simulink model "acs323_m5"  (R2025b)
settings: Solver=ode45  StartTime=0.0  StopTime=300  MaxStep=1  RelTol=1e-3  AbsTol=1e-3  EnableMultiTasking=on
libraries: fuzblock x1, simulink_need_slupdate x1
settings Model: ExtModeTrigMode=oneshot  ExtModeArmWhenConnect=off  Creator=uos  LastModifiedBy=willnatsan
settings SolverCC: AutoScaleAbsTol=off  AlgebraicLoopSolver=TrustRegion
settings DataIOCC: SaveFormat=Array  SignalLoggingSaveFormat=ModelDataLogs  SaveOutput=off  SaveTime=off  ReturnWorkspaceOutputs=off  SignalLoggingName=sigsOut
settings OptimizationCC: BooleanDataType=off  ReuseModelBlockBuffer=off
settings DebuggingCC: SaveWithParameterizedLinksMsg=none  UnderspecifiedInitializationDetection=Classic  MergeDetectMultiDrivingBlocksExec=none  SignalResolutionControl=TryResolveAllWithWarning  MultiTaskDSMMsg=warning  MultiTaskCondExecSysMsg=none  UnconnectedInputMsg=warning  UnconnectedOutputMsg=warning  UnconnectedLineMsg=warning  ArithmeticOperatorsInVariantConditions=warning
settings HardwareCC: ProdBitPerPointer=32.0  ProdBitPerSizeT=32.0  ProdBitPerPtrDiffT=32.0  ProdLargestAtomicFloat=None  ProdIntDivRoundTo=Undefined  ProdEndianess=Unspecified  ProdWordSize=32.0  ProdHWDeviceType=32-bit Generic  TargetUnknown=on
settings ModelReferenceCC: EnableRefExpFcnMdlSchedulingChecks=on  PropagateSignalLabelsOutOfModel=off
settings SFSimCC: SimUseLocalCustomCode=off  CustomCodeUndefinedFunction=UseInterfaceOnly
settings RTWCC: RTWUseLocalCustomCode=off  GPUComputeCapability=3.5  DLArmComputeVersion=19.05
settings GRTTargetCC: TargetLangStandard=C89/C90 (ANSI)  CombineOutputUpdateFcns=off  GRTInterface=on
settings ConfigComp: CovMetricSettings=dw  CovSaveCumulativeToWorkspaceVar=on  CovSaveSingleToWorkspaceVar=on  CovExternalEMLEnable=off

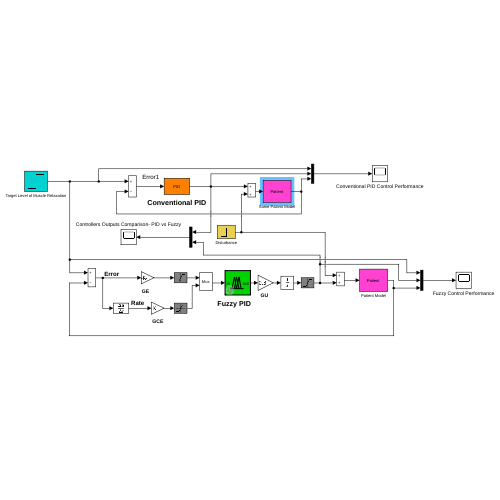
[thumbnail: Simulink's stored preview of the top-level diagram]
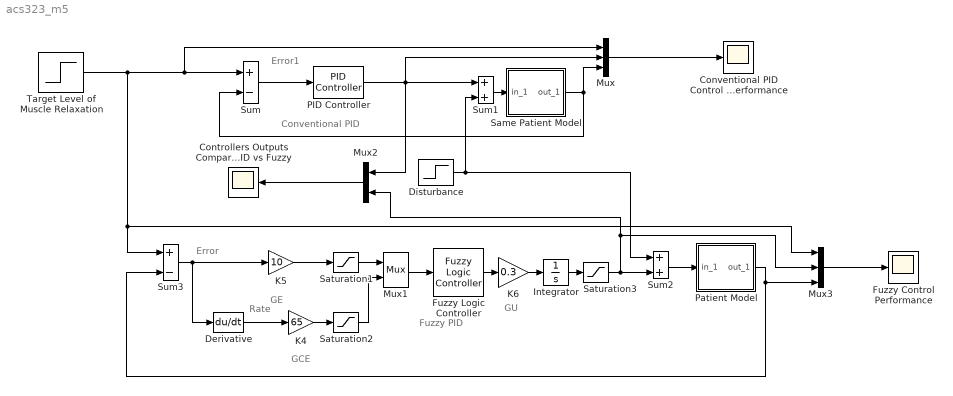
== system acs323_m5 ==
  note: Fuzzy PID
  note: Conventional PID
  note: GE
  note: GCE
  note: GU
  note: Error
  note: Rate
  note: Error1
  Controllers Outputs Comparison- PID vs Fuzzy : Scope
      settings: ActiveDisplayYMinimum=0  ActiveDisplayYMaximum=1.2
  Conventional PID Control Performance : Scope
      settings: ActiveDisplayYMinimum=0.24324  ActiveDisplayYMaximum=0.97781  DataLoggingVariableName=ScopeData2
  Derivative : Derivative
  Disturbance : Step  Time=150  After=0.2  SampleTime=0
  Fuzzy Control Performance : Scope
      settings: ActiveDisplayYMinimum=-0.125  ActiveDisplayYMaximum=1.125
  Fuzzy Logic Controller : fuzblock/Fuzzy Logic  Controller  FIS="\"patient.fis\""  OutputSampleNumber=101  DataType=double  UseLookupTable=off  NumBreakpoints=10  FuzzifiedInputs=off  RuleFiringStrengths=off  RuleOutputs=off  AggregatedOutputs=off  SimulateUsing=Interpreted execution  OutOfRangeInputValueMessage=warning  NoRuleFiredMessage=warning  EmptyOutputFuzzySetMessage=warning
  Integrator : Integrator
  K4 : Gain  Gain=65  SaturateOnIntegerOverflow=on  OutDataTypeStr=Inherit: Same as input  ParamDataTypeStr=Inherit: Same as input
  K5 : Gain  Gain=10  SaturateOnIntegerOverflow=on  OutDataTypeStr=Inherit: Same as input  ParamDataTypeStr=Inherit: Same as input
  K6 : Gain  Gain=0.3  SaturateOnIntegerOverflow=on  OutDataTypeStr=Inherit: Same as input  ParamDataTypeStr=Inherit: Same as input
  Mux : Mux  Inputs=3
  Mux1 : Mux  Inputs=2
  Mux2 : Mux  Inputs=2
  Mux3 : Mux  Inputs=3
  PID Controller : simulink_need_slupdate/PID Controller  P=0.80  I=0.04  D=0
  Patient Model : Subsystem
      mask Display: disp('Patient')
  Same Patient Model : Subsystem
      mask Display: disp('Patient')
  Saturation1 : Saturate  UpperLimit=1  LowerLimit=-1
  Saturation2 : Saturate  UpperLimit=1  LowerLimit=-1
  Saturation3 : Saturate  UpperLimit=1  LowerLimit=0
  Sum : Sum  Inputs=+-  InputSameDT=on  SaturateOnIntegerOverflow=on  OutDataTypeStr=Inherit: Same as first input
  Sum1 : Sum  InputSameDT=on  SaturateOnIntegerOverflow=on  OutDataTypeStr=Inherit: Same as first input
  Sum2 : Sum  InputSameDT=on  SaturateOnIntegerOverflow=on  OutDataTypeStr=Inherit: Same as first input
  Sum3 : Sum  Inputs=+-  InputSameDT=on  SaturateOnIntegerOverflow=on  OutDataTypeStr=Inherit: Same as first input
  Target Level of Muscle Relaxation : Step  Time=0  After=0.8  SampleTime=0
  wires:
  Sum/1 -> PID Controller/1
  Saturation2/1 -> Mux1/2
  Saturation1/1 -> Mux1/1
  Mux1/1 -> Fuzzy Logic Controller/1
  Target Level of Muscle Relaxation/1 -> Sum/1, Mux/1, Mux3/1, Sum3/1
  Sum1/1 -> Same Patient Model/1(in_1)
  Sum2/1 -> Patient Model/1(in_1)
  Saturation3/1 -> Sum2/2, Mux3/2, Mux2/2
  Disturbance/1 -> Sum2/1, Sum1/2
  Mux2/1 -> Controllers Outputs Comparison- PID vs Fuzzy/1
  PID Controller/1 -> Sum1/1, Mux2/1, Mux/2
  Mux/1 -> Conventional PID Control Performance/1
  Mux3/1 -> Fuzzy Control Performance/1
  K4/1 -> Saturation2/1
  Derivative/1 -> K4/1
  Sum3/1 -> K5/1, Derivative/1
  K5/1 -> Saturation1/1
  Patient Model/1(out_1) -> Mux3/3, Sum3/2
  Same Patient Model/1(out_1) -> Sum/2, Mux/3
  K6/1 -> Integrator/1
  Integrator/1 -> Saturation3/1
  Fuzzy Logic Controller/1 -> K6/1

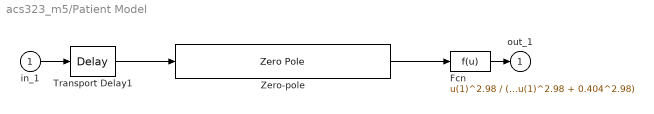
== system acs323_m5/Patient Model ==
  in_1 : Inport
  Fcn : Fcn  Expr=u(1)^2.98 / (u(1)^2.98 + 0.404^2.98)
  Transport Delay1 : TransportDelay
  Zero-pole : ZeroPole  Zeros=[-1/10.64]  Poles=[-1/20.0; -1/3.08; -1/4.81]  Gain=[10.64/(20.0*3.08*4.81)]
  out_1 : Outport  VectorParamsAs1DForOutWhenUnconnected=off
  wires:
  Fcn/1 -> out_1/1
  Zero-pole/1 -> Fcn/1
  in_1/1 -> Transport Delay1/1
  Transport Delay1/1 -> Zero-pole/1

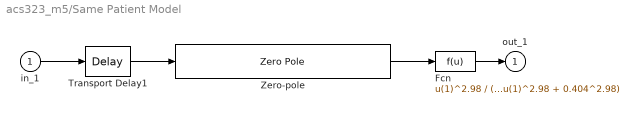
== system acs323_m5/Same Patient Model ==
  in_1 : Inport
  Fcn : Fcn  Expr=u(1)^2.98 / (u(1)^2.98 + 0.404^2.98)
  Transport Delay1 : TransportDelay
  Zero-pole : ZeroPole  Zeros=[-1/10.64]  Poles=[-1/20.0; -1/3.08; -1/4.81]  Gain=[10.64/(20.0*3.08*4.81)]
  out_1 : Outport  VectorParamsAs1DForOutWhenUnconnected=off
  wires:
  Zero-pole/1 -> Fcn/1
  Fcn/1 -> out_1/1
  in_1/1 -> Transport Delay1/1
  Transport Delay1/1 -> Zero-pole/1
